simulink model "rtc_s32k11x"  (Simulink 9.0)
settings: Solver=FixedStepDiscrete  StartTime=0.0  StopTime=10.0  FixedStep=0.1  RelTol=1e-3
InitFcn:
  | mbd_s32k_consistency_checks(bdroot(gcs));
undefined symbols (not defined in the file): LQFP, thumb
libraries: mbd_s32k1xx_ec_toolbox x13, simulink x1
Description:
  | This model demonstrates the "Real Time Clock" functionality by configuring
  | the RTC module to deliver 1Hz Seconds interrupt  and to set an alarm for
  | 5 seconds since the current time.
  | 
  | Validation: When the processor boots up, the RTC is configured. A Seconds
  | ISR was added to toggle the Green LED at 1Hz frecquency. When the SW2
  | button is pressed, it reads the current time and sets the Alarm ISR to be called
  | in the next 5 seconds which will toggle the Blue LED. The time counter is not enabled after
  | initialization done. In order to start the operating mode described above,
  | press the SW3 button.
settings Model: Creator=NXP MBDT Team  LastModifiedBy=nxf35172
settings DataIOCC: ExternalInput=off  InitialState=off  SaveFormat=Dataset  SaveOutput=off  SignalLogging=off  SaveTime=off
settings OptimizationCC: DefaultParameterBehavior=Inlined  PassReuseOutputArgsAs=Individual arguments  LifeSpan=auto
settings DebuggingCC: UnderspecifiedInitializationDetection=Simplified  MergeDetectMultiDrivingBlocksExec=error  InheritedTsInSrcMsg=none  SingleTaskRateTransMsg=error  ParameterTunabilityLossMsg=error  UnconnectedInputMsg=error  UnconnectedOutputMsg=error  UnconnectedLineMsg=error  UnknownTsInhSupMsg=error  SFUnexpectedBacktrackingDiag=error  SFNoUnconditionalDefaultTransitionDiag=error  SFExecutionAtInitializationDiag=warning
settings HardwareCC: ProdLargestAtomicInteger=Long  ProdLargestAtomicFloat=Double  ProdIntDivRoundTo=Zero  ProdEndianess=LittleEndian  ProdHWDeviceType=ARM Compatible->ARM Cortex
settings ModelReferenceCC: PropagateSignalLabelsOutOfModel=on
settings SFSimCC: MATLABDynamicMemAlloc=off
settings RTWCC: SystemTargetFile=mbd_s32k.tlc  MakeCommand=mbd_s32k_make_rtw COPY_MDLREF_INCLUDES=0  TemplateMakefile=mbd_s32k.tmf  Description=Model Based Design Toolbox S32K11x Code Generation Target  GenerateReport=on  IncludeHyperlinkInReport=on  LaunchReport=on  GenerateTraceInfo=on  GenerateTraceReport=on  GenerateTraceReportSl=on  GenerateTraceReportSf=on  GenerateTraceReportEml=on
settings CodeAppCC: ForceParamTrailComments=on  IgnoreCustomStorageClasses=off  OperatorAnnotations=on  SimulinkDataObjDesc=on  SFDataObjDesc=on  InsertBlockDesc=on  StateflowObjectComments=off
settings STFCustomTargetCC: TargetLangStandard=C99 (ISO)  MultiwordLength=256  CombineOutputUpdateFcns=on  ERTCustomFileBanners=on  SupportContinuousTime=off  SupportNonInlinedSFcns=off  RemoveResetFunc=on  MATLABClassNameForMDSCustomization=Simulink.SoftwareTarget.ERTCustomization  GRTInterface=off  SystemTargetFile=mbd_s32k11.tlc
settings ERTTargetCC: TargetLangStandard=C99 (ISO)  ParMdlRefBuildCompliant=off  CompOptLevelCompliant=off  ConcurrentExecutionCompliant=off  ModelStepFunctionPrototypeControlCompliant=off  CPPClassGenCompliant=off  UseToolchainInfoCompliant=off  InlinedParameterPlacement=NonHierarchical  ERTSrcFileBannerTemplate=mbd_ert_code_template.cgt  ERTHdrFileBannerTemplate=mbd_ert_code_template.cgt  ERTDataSrcFileTemplate=mbd_ert_code_template.cgt  ERTDataHdrFileTemplate=mbd_ert_code_template.cgt  ERTCustomFileTemplate=example_file_process.tlc
settings ConfigComp: CovMetricSettings=dwe  CovHtmlReporting=off  CovSaveCumulativeToWorkspaceVar=off  CovSaveSingleToWorkspaceVar=off  CovExternalEMLEnable=on

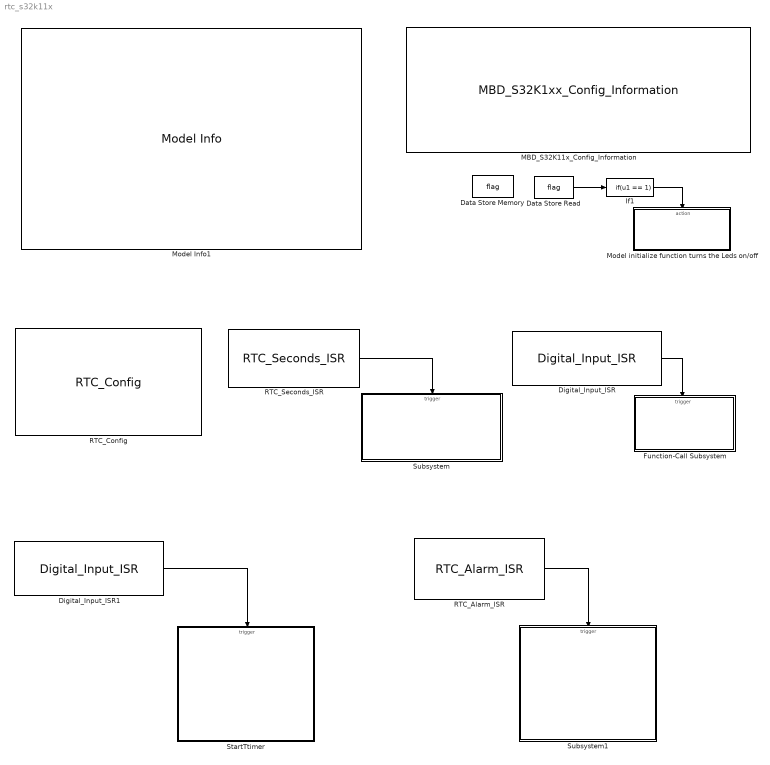
== system rtc_s32k11x ==
  Data Store Memory : DataStoreMemory  DataStoreName=flag  ReadBeforeWriteMsg=warning  WriteAfterWriteMsg=warning  WriteAfterReadMsg=warning  InitialValue=1  ShowAdditionalParam=off  OutDataTypeStr=boolean
  Data Store Read : DataStoreRead  DataStoreName=flag
  Digital_Input_ISR : mbd_s32k1xx_ec_toolbox/GPIO Blocks/Digital_Input_ISR  gpio_pin=PTD3: [PTD3 | Port D I/O]  irqc=on rising-edge  prio=2
  Digital_Input_ISR1 : mbd_s32k1xx_ec_toolbox/GPIO Blocks/Digital_Input_ISR  gpio_pin=PTD5: [PTD5 | Port D I/O]  irqc=on rising-edge  prio=5
  Function-Call Subsystem : Subsystem  TreatAsAtomicUnit=on
  If1 : If  IfExpression=u1 == 1  ShowElse=off
  MBD_S32K11x_Config_Information : mbd_s32k1xx_ec_toolbox/MBD_S32K1xx_Config_Information  mbdt_ver=0  disp_str=|  config_params=[]  mcu_target_name=S32K118  mcu_target_package=64-LQFP  mcu_target_sram_size=25KB  mcu_system_clock_freq=40  mcu_xtal_freq=External 40  mcu_steptick_timer=LPIT Channel 0  mcu_steptick_prio=3  ds_import_enable=on  target_compiler=GCC  target_memory=FLASH  gcc_target_compile_opts=-mcpu=cortex-m0plus -mthumb -O1 -g -gstrict-dwarf  gcc_target_assemble_opts=-mcpu=cortex-m0plus -mthumb -g  gcc_target_link_opts=-mcpu=cortex-m0plus -mthumb  gcc_target_default_lcf=on  gcc_target_user_lcf=S32K118_25_flash.ld  ghs_target_compile_opts=-mcpu=cortexm0plus -mthumb -fsoft -Ogeneral -Wundef -Wimplicit-int -Wshadow -Wtrigraphs --no_commons --gnu_asm -gnu99 -gdwarf-2 -G  ghs_target_assemble_opts=-mcpu=cortexm0plus -mthumb -fsoft --gnu_asm  ghs_target_link_opts=-mcpu=cortexm0plus -mthumb -fsoft  ghs_target_default_lcf=on  ghs_target_user_lcf=S32K118_25_flash.ld  iar_target_compile_opts=--thumb -Ol -e --debug --dlib_config normal  iar_target_assemble_opts=--thumb  iar_target_link_opts=--no_exceptions --vfe --inline  iar_target_default_lcf=on  iar_target_user_lcf=S32K118_25_flash.icf  pil_download_enable=off  rbl_download_enable=on  rbl_start_delay=5000  rbl_download_interface=OpenSDA  rbl_restart_request=off  rbl_com_port=Custom  rbl_com_port_custom=COM1  pil_download_rate=57600  pil_opensda_drive=Custom  pil_opensda_drive_custom=D  pil_uart_instance=0  pil_uart_rx=PTA2: [LPUART0_RX | Receive]  pil_uart_tx=PTA3: [LPUART0_TX | Transmit]  FTM_PWM_PcrCheckEnDis=on  FTM_Input_Edge_Inputs_PcrCheckEnDis=on  FTM_Dual_Edge_Inputs_PcrCheckEnDis=on  FTM_Quadrature_Inputs_PcrCheckEnDis=on  FTM_Hall_Sensor_Inputs_PcrCheckEnDis=on  LPTMR_PcrCheckEnDis=on  PIT_PcrCheckEnDis=on  RTC_PcrCheckEnDis=on  FlexCAN_PcrCheckEnDis=on  LIN_PcrCheckEnDis=on  FlexIO_PcrCheckEnDis=on  LPI2C_PcrCheckEnDis=on  LPSPI_PcrCheckEnDis=on  LPUART_PcrCheckEnDis=on  CMP_PcrCheckEnDis=on  GPIO_OutputPcrCheckEnDis=on  GPIO_InputPcrCheckEnDis=on  SBC_PcrCheckEnDis=on  AMMCLIB_PcrCheckEnDis=on  FM_PcrCheckEnDis=on  Profile_PcrCheckEnDis=on  ConfigParams_PcrCheckEnDis=on  ModelRef_PcrCheckEnDis=on  PDB0_PcrCheckEnDis=on  CSEc_PcrCheckEnDis=on  eDMA_PcrCheckEnDis=on  ADC_PcrCheckEnDis=on  WDOG_PcrCheckEnDis=on
      | Target : S32K144-64KB_SRAM
      | Package : 100-pin
      | System clock : 80 MHz
      | XTAL clock : External 8 MHz
      | Compiler : IAR
      | Target Type : FLASH
      | Download Code after build : off
      | Step Tick Interrupt Priority : 15
  Model Info1 : simulink/Model-Wide Utilities/Model Info  Frame=off  DisplayStringWithTags=|  HorizontalTextAlignment=Left  LeftAlignmentValue=0.02
      | Model Name: %<ModelName>
      | 
      | Description: %<Description>
  Model initialize function turns the Leds on/off : Subsystem
  RTC_Alarm_ISR : mbd_s32k1xx_ec_toolbox/Core and System Blocks/RTC Blocks/RTC_Alarm_ISR  Priority=1
  RTC_Config : mbd_s32k1xx_ec_toolbox/Core and System Blocks/RTC Blocks/RTC_Config  Priority=2  date_day=1  date_month=1  date_year=1970  time_hour=0  time_min=0  time_sec=0  show_adv_opts=on  clock_input=1KHz LPO  clock_output=Disabled  comp_state=off  comp_value=0  comp_interval=0  state_update=off  state_w_access=off  state_read_only=off  start_counter=off
  RTC_Seconds_ISR : mbd_s32k1xx_ec_toolbox/Core and System Blocks/RTC Blocks/RTC_Seconds_ISR  sec_irq_freq=1Hz
  StartTtimer : Subsystem
  Subsystem : Subsystem
  Subsystem1 : Subsystem
  wires:
  Data Store Read/1 -> If1/1
  Digital_Input_ISR1/1 -> StartTtimer/Trigger
  RTC_Alarm_ISR/1 -> Subsystem1/Trigger
  RTC_Seconds_ISR/1 -> Subsystem/Trigger
  Digital_Input_ISR/1 -> Function-Call Subsystem/Trigger
  If1/1 -> Model initialize function turns the Leds on/off/Action

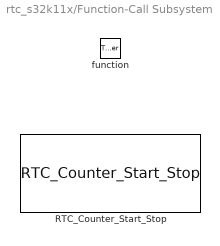
== system rtc_s32k11x/Function-Call Subsystem ==
  function : TriggerPort  TriggerType=function-call  VariantControl=Variant
  RTC_Counter_Start_Stop : mbd_s32k1xx_ec_toolbox/Core and System Blocks/RTC Blocks/RTC_Counter_Start_Stop  set_action=Start

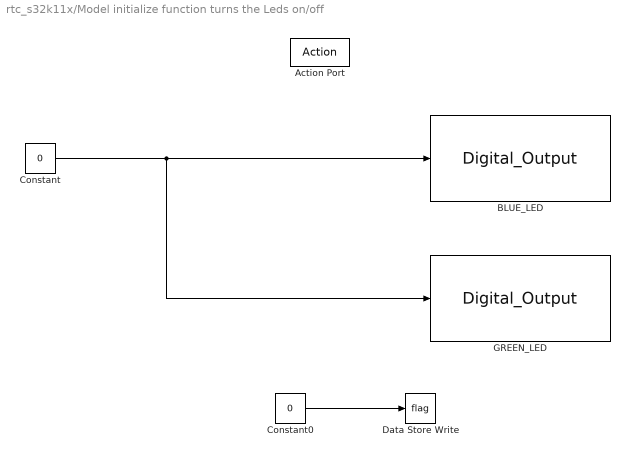
== system rtc_s32k11x/Model initialize function turns the Leds on/off ==
  Action Port : ActionPort
  BLUE_LED : mbd_s32k1xx_ec_toolbox/GPIO Blocks/Digital_Output  gpio_pin=PTE8: [PTE8 | Port E I/O]  init_val=Low  drive_strength=High
  Constant : Constant  Value=0  OutDataTypeStr=boolean
  Constant0 : Constant  Value=0  OutDataTypeStr=boolean
  Data Store Write : DataStoreWrite  DataStoreName=flag
  GREEN_LED : mbd_s32k1xx_ec_toolbox/GPIO Blocks/Digital_Output  gpio_pin=PTD15: [PTD15 | Port D I/O]  init_val=Low  drive_strength=Low
  wires:
  Constant/1 -> GREEN_LED/1, BLUE_LED/1
  Constant0/1 -> Data Store Write/1

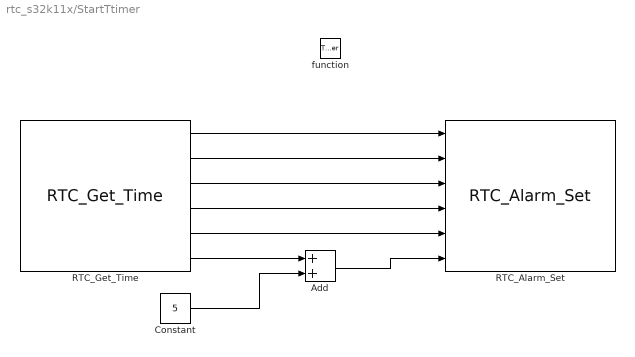
== system rtc_s32k11x/StartTtimer ==
  function : TriggerPort  TriggerType=function-call  VariantControl=Variant
  Add : Sum  Priority=2
  Constant : Constant  Value=5  OutDataTypeStr=uint8
  RTC_Alarm_Set : mbd_s32k1xx_ec_toolbox/Core and System Blocks/RTC Blocks/RTC_Alarm_Set  Priority=3  inputs_enable=on  date_day=1  date_month=1  date_year=1970  time_hour=0  time_min=0  time_sec=0  show_adv_opts=on  repeat=off  interval=5  forever=on  repeats=0
  RTC_Get_Time : mbd_s32k1xx_ec_toolbox/Core and System Blocks/RTC Blocks/RTC_Get_Time  Priority=1
  wires:
  RTC_Get_Time/1 -> RTC_Alarm_Set/1
  RTC_Get_Time/2 -> RTC_Alarm_Set/2
  RTC_Get_Time/3 -> RTC_Alarm_Set/3
  RTC_Get_Time/4 -> RTC_Alarm_Set/4
  RTC_Get_Time/5 -> RTC_Alarm_Set/5
  RTC_Get_Time/6 -> Add/1
  Add/1 -> RTC_Alarm_Set/6
  Constant/1 -> Add/2

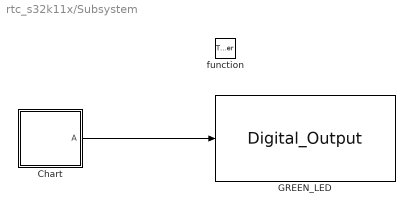
== system rtc_s32k11x/Subsystem ==
  function : TriggerPort  TriggerType=function-call  VariantControl=Variant
  Chart : Stateflow chart  TreatAsAtomicUnit=on
  GREEN_LED : mbd_s32k1xx_ec_toolbox/GPIO Blocks/Digital_Output  gpio_pin=PTD15: [PTD15 | Port D I/O]  init_val=Low  drive_strength=Low
  wires:
  Chart/1(" A") -> GREEN_LED/1

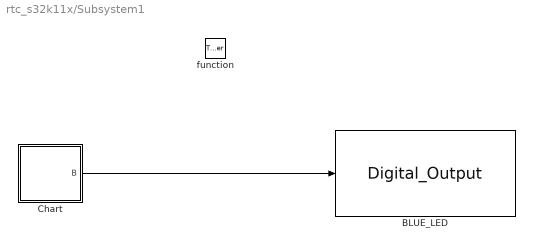
== system rtc_s32k11x/Subsystem1 ==
  function : TriggerPort  TriggerType=function-call  VariantControl=Variant
  BLUE_LED : mbd_s32k1xx_ec_toolbox/GPIO Blocks/Digital_Output  gpio_pin=PTE8: [PTE8 | Port E I/O]  init_val=Low  drive_strength=High
  Chart : Stateflow chart  TreatAsAtomicUnit=on
  wires:
  Chart/1(" B") -> BLUE_LED/1

== stateflow chart Subsystem1/Chart ==
  state B
  state B1
  (default) -> B
  B -> B1
  B1 -> B
  data: B output boolean [0..1]

== stateflow chart Subsystem/Chart ==
  state A
  state A1
  (default) -> A
  A -> A1
  A1 -> A
  data: A output boolean [0..1]
